simulink model "Target_Control_System"  (R2021b)
settings: Solver=FixedStepDiscrete  StartTime=0.0  StopTime=5  RelTol=1e-3
PreLoadFcn:
  | RTWConfigurationCB('preloadfcn', bdroot);
PostLoadFcn:
  | load('configuration/data_struct.mat');
  | load('configuration/fluxMaps_propMotor.mat');
  | load('configuration/parameterInit_PROP.mat');
  | load('configuration/parameterInit_PUMP.mat');
  | load('configuration/parameterInit_PITCH.mat');
  | load('configuration/parameterInit_TILT.mat');
  | %load('configuration/base_workspace_signal_definition.mat');
  | %load('resolvedatastores_to_baseworkspace_for_faster_simulation.mat');
model workspace (MAT data in the model file):
  SIMULATION_OPTIONS : Simulink.Parameter (value not decoded)
  TARGET_CODE_GEN : Simulink.Parameter (value not decoded)
  TCS_SAMPLE_FREQ_HZ : Simulink.Parameter (value not decoded)
symbols that are objects in the model workspace (value not decoded): TARGET_CODE_GEN, TCS_SAMPLE_FREQ_HZ
undefined symbols (not defined in the file): A_DQ_REF_LPF_INIT__PITCH, A_DQ_REF_LPF_INIT__PROP, A_DQ_REF_LPF_INIT__PUMP, A_DQ_REF_LPF_INIT__TILT, A_OBSERVER_CONFIDENCE_INIT__PITCH, A_OBSERVER_CONFIDENCE_INIT__PROP, A_OBSERVER_CONFIDENCE_INIT__PUMP, A_OBSERVER_CONFIDENCE_INIT__TILT, ACTUATOR_MAX_ANGLE_TRIP__PITCH, ACTUATOR_MIN_ANGLE_TRIP__PITCH, ACTUATOR_POS_SENSOR_INV_DIRECTION__PITCH, ACTUATOR_POS_SENSOR_INV_DIRECTION__TILT, ACTUATOR_POS_SENSOR_OFFSET__PITCH, ACTUATOR_POS_SENSOR_OFFSET__TILT, ADC_scaler1_baseaddr_TILT, ADC_SCALER_FLOAT_TO_FIXPOINT_EXPANSION, ANGLE_ELEC_FROM_SENSOR_OFFSET_INIT__PITCH, ANGLE_ELEC_FROM_SENSOR_OFFSET_INIT__PROP, ANGLE_ELEC_FROM_SENSOR_OFFSET_INIT__PUMP, ANGLE_ELEC_FROM_SENSOR_OFFSET_INIT__TILT, AUTO_CLEAR_FAULTS_ENABLED__PITCH, AUTO_CLEAR_FAULTS_ENABLED__PROP, AUTO_CLEAR_FAULTS_ENABLED__PUMP, AUTO_CLEAR_FAULTS_ENABLED__TILT, AUTO_CLEAR_FAULTS_WAIT_TICKS__PITCH, AUTO_CLEAR_FAULTS_WAIT_TICKS__PROP, AUTO_CLEAR_FAULTS_WAIT_TICKS__PUMP, AUTO_CLEAR_FAULTS_WAIT_TICKS__TILT, AUTO_I_ZERO_IDLE_TICKS__PITCH, AUTO_I_ZERO_IDLE_TICKS__PROP, AUTO_I_ZERO_IDLE_TICKS__PUMP, AUTO_I_ZERO_IDLE_TICKS__TILT, AUTO_I_ZERO_OFFSET_IDC_THRESHOLD__PITCH, AUTO_I_ZERO_OFFSET_IDC_THRESHOLD__PROP, AUTO_I_ZERO_OFFSET_IDC_THRESHOLD__PUMP, AUTO_I_ZERO_OFFSET_IDC_THRESHOLD__TILT, AUTO_I_ZERO_OFFSET_IPH_THRESHOLD__PITCH, AUTO_I_ZERO_OFFSET_IPH_THRESHOLD__PROP, AUTO_I_ZERO_OFFSET_IPH_THRESHOLD__PUMP, AUTO_I_ZERO_OFFSET_IPH_THRESHOLD__TILT, AUTO_SENSORLESS_SWITCHOVER_DISABLE_OMEGA, AUTO_SENSORLESS_SWITCHOVER_ENABLE_OMEGA, AUTO_SENSORLESS_SWITCHOVER_MIN_CONFIDENCE, AUXILIARY_PROTECTION_UNIT_BASEADDR__TILT, blanking_max_error_omega_INIT_PITCH, blanking_max_error_omega_INIT_TILT, blanking_max_error_position_INIT_PITCH, blanking_max_error_position_INIT_TILT, BRUTE_START_I_Q_REF_RAMP_SPEED__PITCH, BRUTE_START_I_Q_REF_RAMP_SPEED__PROP, BRUTE_START_I_Q_REF_RAMP_SPEED__PUMP, BRUTE_START_I_Q_REF_RAMP_SPEED__TILT, CONTROL_LOOP_DT_INIT__PITCH, CONTROL_LOOP_DT_INIT__PROP, CONTROL_LOOP_DT_INIT__PUMP, CONTROL_LOOP_DT_INIT__TILT, CORRECTION_FILTER_SCALE__PITCH, CORRECTION_FILTER_SCALE__PROP, CORRECTION_FILTER_SCALE__PUMP, CORRECTION_FILTER_SCALE__TILT ... (+458)
libraries: simulink x178, Reusables_Lib x24
(part 18 of 47)

== system Target_Control_System/Target_Control_System/Simulation Controls/Simulation Data Store Initialization/initializeDataForTilt()/initializeHardwareInvTilt ==
  initializeHardwareInvTilt : TriggerPort  TriggerType=function-call  VariantControl=Variant
  Constant : Constant  Value=4.0  OutDataTypeStr=single
  Constant1 : Constant  Value=DEADTIME_NS__TILT  OutDataTypeStr=single
  Constant10 : Constant  Value=VOLTAGE_OFFSET_DC_V_JULY2019__TILT  OutDataTypeStr=single
  Constant11 : Constant  Value=FULL_SCALE_VALUE_DC_VOLTAGE_V_JULY2019__TILT  OutDataTypeStr=single
  Constant12 : Constant  Value=ADC_SCALER_FLOAT_TO_FIXPOINT_EXPANSION  OutDataTypeStr=single
  Constant13 : Constant  Value=PHASE_CURRENT_SUM_MAX_IMBALANCE__TILT  OutDataTypeStr=single
  Constant14 : Constant  Value=MAX_IDENTICAL_SAMPLES_PHASE_CURRENT__TILT  OutDataTypeStr=int32
  Constant15 : Constant  Value=AUXILIARY_PROTECTION_UNIT_BASEADDR__TILT  OutDataTypeStr=uint32
  Constant16 : Constant  Commented=on  Value=GateDriver_baseaddr_TILT  OutDataTypeStr=single
  Constant17 : Constant  Commented=on  Value=ADC_scaler1_baseaddr_TILT  OutDataTypeStr=single
  Constant18 : Constant  Commented=on  Value=PWM1_baseaddr_TILT  OutDataTypeStr=single
  Constant19 : Constant  Commented=on  Value=IIR_baseaddr_TILT  OutDataTypeStr=single
  Constant2 : Constant  Value=IIR_DC_F_INIT__TILT  OutDataTypeStr=single
  Constant21 : Constant  Commented=on  Value=TILT_INPUT_ENCODER_base_addr  OutDataTypeStr=single
  Constant22 : Constant  Commented=on  Value=TILT_OUTPUT_ENCODER_base_addr  OutDataTypeStr=single
  Constant3 : Constant  Value=IIR_UPHASE_F_INIT__TILT  OutDataTypeStr=single
  Constant4 : Constant  Value=IIR_IPHASE_F_INIT__TILT  OutDataTypeStr=single
  Constant5 : Constant  Value=IIR_F_SAMPLE__TILT  OutDataTypeStr=single
  Constant6 : Constant  Value=FULL_SCALE_VALUE_PHASE_VOLTAGE_V__TILT  OutDataTypeStr=single
  Constant7 : Constant  Value=FULL_SCALE_VALUE_PHASE_CURRENT_A__TILT  OutDataTypeStr=single
  Constant8 : Constant  Value=FULL_SCALE_VALUE_DC_CURRENT_A__TILT  OutDataTypeStr=single
  Constant9 : Constant  Value=VOLTAGE_OFFSET_V__TILT  OutDataTypeStr=single
  Data Store Write : DataStoreWrite  DataStoreName=oTilt  DataStoreElements=oTilt.oHw_.fTripLimitHardware_  IndexOptions=Index vector (dialog)  Indices=1  OutputSizes=1
  Data Store Write1 : DataStoreWrite  DataStoreName=oTilt  DataStoreElements=oTilt.oHw_.fDeadtimeNs_  IndexOptions=Index vector (dialog)  Indices=1  OutputSizes=1
  Data Store Write10 : DataStoreWrite  DataStoreName=oTilt  DataStoreElements=oTilt.oHw_.fFullScaleValueDcVoltage_  IndexOptions=Index vector (dialog)  Indices=1  OutputSizes=1
  Data Store Write11 : DataStoreWrite  DataStoreName=oTilt  DataStoreElements=oTilt.oHw_.fVoltageOffsetDcInVolts_  IndexOptions=Index vector (dialog)  Indices=1  OutputSizes=1
  Data Store Write12 : DataStoreWrite  DataStoreName=oTilt  DataStoreElements=oTilt.oHw_.iScalePhaseCurrentLong_  IndexOptions=Index vector (dialog)  Indices=1  OutputSizes=1
  Data Store Write13 : DataStoreWrite  DataStoreName=oTilt  DataStoreElements=oTilt.oHw_.iScaleDcCurrentLong_  IndexOptions=Index vector (dialog)  Indices=1  OutputSizes=1
  Data Store Write14 : DataStoreWrite  DataStoreName=oTilt  DataStoreElements=oTilt.oHw_.iScalePhaseVoltageLong_  IndexOptions=Index vector (dialog)  Indices=1  OutputSizes=1
  Data Store Write15 : DataStoreWrite  DataStoreName=oTilt  DataStoreElements=oTilt.oHw_.iScaleDcVoltageLong_  IndexOptions=Index vector (dialog)  Indices=1  OutputSizes=1
  Data Store Write16 : DataStoreWrite  DataStoreName=oTilt  DataStoreElements=oTilt.oHw_.fPhaseCurrentSumMaxImbalance_  IndexOptions=Index vector (dialog)  Indices=1  OutputSizes=1
  Data Store Write17 : DataStoreWrite  DataStoreName=oTilt  DataStoreElements=oTilt.oHw_.iMaxIdenticalSamplesPhaseCurrent_  IndexOptions=Index vector (dialog)  Indices=1  OutputSizes=1
  Data Store Write18 : DataStoreWrite  DataStoreName=oTilt  DataStoreElements=oTilt.oHw_.uiAuxiliaryProtectionUnitBaseaddr_  IndexOptions=Index vector (dialog)  Indices=1  OutputSizes=1
  Data Store Write19 : DataStoreWrite  DataStoreName=oTilt  DataStoreElements=oTilt.oHw_.iVoltageOffsetPhsLong_  IndexOptions=Index vector (dialog)  Indices=1  OutputSizes=1
  Data Store Write2 : DataStoreWrite  DataStoreName=oTilt  DataStoreElements=oTilt.oHw_.fIirDcFInit_  IndexOptions=Index vector (dialog)  Indices=1  OutputSizes=1
  Data Store Write20 : DataStoreWrite  DataStoreName=oTilt  DataStoreElements=oTilt.oHw_.iVoltageOffsetDcLong_  IndexOptions=Index vector (dialog)  Indices=1  OutputSizes=1
  Data Store Write21 : DataStoreWrite  Commented=on  DataStoreName=oTilt  DataStoreElements=oTilt.oHw_.uiPwmGeneratorBaseaddr_  IndexOptions=Index vector (dialog)  Indices=1  OutputSizes=1
  Data Store Write22 : DataStoreWrite  Commented=on  DataStoreName=oTilt  DataStoreElements=oTilt.oHw_.uiIirInterfaceBaseaddr_  IndexOptions=Index vector (dialog)  Indices=1  OutputSizes=1
  Data Store Write23 : DataStoreWrite  Commented=on  DataStoreName=oTilt  DataStoreElements=oTilt.oHw_.uiInputPositionSensorBaseaddr_  IndexOptions=Index vector (dialog)  Indices=1  OutputSizes=1
  Data Store Write24 : DataStoreWrite  Commented=on  DataStoreName=oTilt  DataStoreElements=oTilt.oHw_.uiOutputPositionSensorBaseaddr_  IndexOptions=Index vector (dialog)  Indices=1  OutputSizes=1
  Data Store Write26 : DataStoreWrite  Commented=on  DataStoreName=oTilt  DataStoreElements=oTilt.oHw_.uiGateDriverBaseaddr_  IndexOptions=Index vector (dialog)  Indices=1  OutputSizes=1
  Data Store Write27 : DataStoreWrite  Commented=on  DataStoreName=oTilt  DataStoreElements=oTilt.oHw_.uiAdcScalerBaseaddr_  IndexOptions=Index vector (dialog)  Indices=1  OutputSizes=1
  Data Store Write3 : DataStoreWrite  DataStoreName=oTilt  DataStoreElements=oTilt.oHw_.fIirUphaseFInit_  IndexOptions=Index vector (dialog)  Indices=1  OutputSizes=1
  Data Store Write4 : DataStoreWrite  DataStoreName=oTilt  DataStoreElements=oTilt.oHw_.fIirIphaseFInit_  IndexOptions=Index vector (dialog)  Indices=1  OutputSizes=1
  Data Store Write5 : DataStoreWrite  DataStoreName=oTilt  DataStoreElements=oTilt.oHw_.fIirFSample_  IndexOptions=Index vector (dialog)  Indices=1  OutputSizes=1
  Data Store Write6 : DataStoreWrite  DataStoreName=oTilt  DataStoreElements=oTilt.oHw_.fFullScaleValuePhaseCurrent_  IndexOptions=Index vector (dialog)  Indices=1  OutputSizes=1
  Data Store Write7 : DataStoreWrite  DataStoreName=oTilt  DataStoreElements=oTilt.oHw_.fFullScaleValueDcCurrent_  IndexOptions=Index vector (dialog)  Indices=1  OutputSizes=1
  Data Store Write8 : DataStoreWrite  DataStoreName=oTilt  DataStoreElements=oTilt.oHw_.fFullScaleValuePhaseVoltage_  IndexOptions=Index vector (dialog)  Indices=1  OutputSizes=1
  Data Store Write9 : DataStoreWrite  DataStoreName=oTilt  DataStoreElements=oTilt.oHw_.fVoltageOffsetInVolts_  IndexOptions=Index vector (dialog)  Indices=1  OutputSizes=1
  Divide{,1..5} (6 alike) : Product  Inputs=**  OutDataTypeStr=int32
  wires:
  Divide1/1 -> Data Store Write12/1
  Divide/1 -> Data Store Write13/1
  Constant10/1 -> Data Store Write11/1, Divide5/1
  Divide5/1 -> Data Store Write20/1
  Divide4/1 -> Data Store Write19/1
  Constant9/1 -> Data Store Write9/1, Divide4/1
  Constant22/1 -> Data Store Write24/1
  Constant4/1 -> Data Store Write4/1
  Constant3/1 -> Data Store Write3/1
  Constant2/1 -> Data Store Write2/1
  Constant17/1 -> Data Store Write27/1
  Constant8/1 -> Data Store Write7/1, Divide/1
  Divide2/1 -> Data Store Write14/1
  Divide3/1 -> Data Store Write15/1
  Constant1/1 -> Data Store Write1/1
  Constant11/1 -> Data Store Write10/1, Divide3/1
  Constant15/1 -> Data Store Write18/1
  Constant5/1 -> Data Store Write5/1
  Constant6/1 -> Data Store Write8/1, Divide2/1
  Constant14/1 -> Data Store Write17/1
  Constant19/1 -> Data Store Write22/1
  Constant/1 -> Data Store Write/1
  Constant18/1 -> Data Store Write21/1
  Constant16/1 -> Data Store Write26/1
  Constant12/1 -> Divide/2, Divide5/2, Divide3/2, Divide4/2, Divide2/2, Divide1/2
  Constant13/1 -> Data Store Write16/1
  Constant21/1 -> Data Store Write23/1
  Constant7/1 -> Data Store Write6/1, Divide1/1

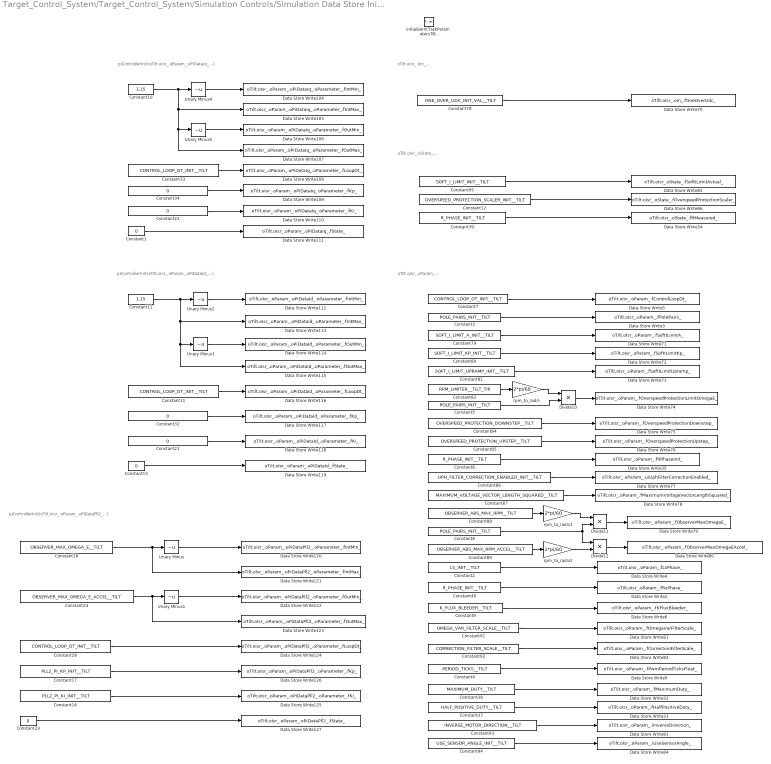
== system Target_Control_System/Target_Control_System/Simulation Controls/Simulation Data Store Initialization/initializeDataForTilt()/initializeIntTaskParametersTilt ==
  note: oTilt.oIsr_.oState_...
  note: oTilt.oIsr_.oParam_...
  note: oTilt.oIsr_.oIn_...
  note: piControllerInit(oTilt.oIsr_.oParam_.oPiDataIq_...)
  note: piControllerInit(oTilt.oIsr_.oParam_.oPiDataPll2_...)
  note: piControllerInit(oTilt.oIsr_.oParam_.oPiDataId_...)
  initializeIntTaskParametersTilt : TriggerPort  TriggerType=function-call  VariantControl=Variant
  Constant{1,15,21..22,32,34} (6 alike) : Constant  Value=0  OutDataTypeStr=single  SampleTime=-1
  Constant10 : Constant  Value=1.15  OutDataTypeStr=single  SampleTime=-1
  Constant11 : Constant  Value=1.15  OutDataTypeStr=single  SampleTime=-1
  Constant12 : Constant  Value=OVERSPEED_PROTECTION_SCALER_INIT__TILT  OutDataTypeStr=single  SampleTime=-1
  Constant16 : Constant  Value=PLL2_PI_KI_INIT__TILT  OutDataTypeStr=single  SampleTime=-1
  Constant17 : Constant  Value=PLL2_PI_KP_INIT__TILT  OutDataTypeStr=single  SampleTime=-1
  Constant18 : Constant  Value=OBSERVER_MAX_OMEGA_E__TILT  OutDataTypeStr=single  SampleTime=-1
  Constant2 : Constant  Value=LS_INIT__TILT  OutDataTypeStr=single  SampleTime=-1
  Constant23 : Constant  Value=0  OutDataTypeStr=single
  Constant24 : Constant  Value=OBSERVER_MAX_OMEGA_E_ACCEL__TILT  OutDataTypeStr=single  SampleTime=-1
  Constant28 : Constant  Value=CONTROL_LOOP_DT_INIT__TILT  OutDataTypeStr=single  SampleTime=-1
  Constant3 : Constant  Value=POLE_PAIRS_INIT__TILT  VectorParams1D=off  OutDataTypeStr=single  SampleTime=-1
  Constant31 : Constant  Value=CONTROL_LOOP_DT_INIT__TILT  OutDataTypeStr=single  SampleTime=-1
  Constant33 : Constant  Value=CONTROL_LOOP_DT_INIT__TILT  OutDataTypeStr=single  SampleTime=-1
  Constant37 : Constant  Value=HALF_POSITIVE_DUTY__TILT  OutDataTypeStr=single  SampleTime=-1
  Constant38 : Constant  Value=MAXIMUM_DUTY__TILT  OutDataTypeStr=single  SampleTime=-1
  Constant39 : Constant  Value=R_PHASE_INIT__TILT  OutDataTypeStr=single  SampleTime=-1
  Constant4 : Constant  Value=PERIOD_TICKS__TILT  OutDataTypeStr=single  SampleTime=-1
  Constant40 : Constant  Value=R_PHASE_INIT__TILT  OutDataTypeStr=single  SampleTime=-1
  Constant5 : Constant  Value=POLE_PAIRS_INIT__TILT  VectorParams1D=off  OutDataTypeStr=single  SampleTime=-1
  Constant6 : Constant  Value=R_PHASE_INIT__TILT  VectorParams1D=off  OutDataTypeStr=single  SampleTime=-1
  Constant7 : Constant  Value=CONTROL_LOOP_DT_INIT__TILT  VectorParams1D=off  OutDataTypeStr=single  SampleTime=-1
  Constant78 : Constant  Value=ONE_OVER_UDC_INIT_VAL__TILT  VectorParams1D=off  OutDataTypeStr=single  SampleTime=-1
  Constant79 : Constant  Value=SOFT_I_LIMIT_A_INIT__TILT  OutDataTypeStr=single  SampleTime=-1
  Constant8 : Constant  Value=POLE_PAIRS_INIT__TILT  VectorParams1D=off  OutDataTypeStr=single  SampleTime=-1
  Constant80 : Constant  Value=SOFT_I_LIMIT_KP_INIT__TILT  OutDataTypeStr=single  SampleTime=-1
  Constant81 : Constant  Value=SOFT_I_LIMIT_UPRAMP_INIT__TILT  OutDataTypeStr=single  SampleTime=-1
  Constant82 : Constant  Value=RPM_LIMITER__TILT_TIP  OutDataTypeStr=single  SampleTime=-1
  Constant84 : Constant  Value=OVERSPEED_PROTECTION_DOWNSTEP__TILT  OutDataTypeStr=single  SampleTime=-1
  Constant85 : Constant  Value=OVERSPEED_PROTECTION_UPSTEP__TILT  OutDataTypeStr=single  SampleTime=-1
  Constant86 : Constant  Value=UPH_FILTER_CORRECTION_ENABLED_INIT__TILT  OutDataTypeStr=uint32  SampleTime=-1
  Constant87 : Constant  Value=MAXIMUM_VOLTAGE_VECTOR_LENGTH_SQUARED__TILT  VectorParams1D=off  OutDataTypeStr=single  SampleTime=-1
  Constant88 : Constant  Value=OBSERVER_ABS_MAX_RPM__TILT  OutDataTypeStr=single  SampleTime=-1
  Constant89 : Constant  Value=OBSERVER_ABS_MAX_RPM_ACCEL__TILT  OutDataTypeStr=single  SampleTime=-1
  Constant9 : Constant  Value=K_FLUX_BLEEDER__TILT  VectorParams1D=off  OutDataTypeStr=single  SampleTime=-1
  Constant91 : Constant  Value=OMEGA_VAR_FILTER_SCALE__TILT  OutDataTypeStr=single  SampleTime=-1
  Constant92 : Constant  Value=CORRECTION_FILTER_SCALE__TILT  OutDataTypeStr=single  SampleTime=-1
  Constant93 : Constant  Value=INVERSE_MOTOR_DIRECTION__TILT  OutDataTypeStr=int32  SampleTime=-1
  Constant94 : Constant  Value=USE_SENSOR_ANGLE_INIT__TILT  OutDataTypeStr=int32  SampleTime=-1
  Constant95 : Constant  Value=SOFT_I_LIMIT_INIT__TILT  OutDataTypeStr=single  SampleTime=-1
  Data Store Write104 : DataStoreWrite  DataStoreName=oTilt  DataStoreElements=oTilt.oIsr_.oParam_.oPiDataIq_.oParameter_.fIntMin_  IndexOptions=Index vector (dialog)  Indices=1  OutputSizes=1
  Data Store Write105 : DataStoreWrite  DataStoreName=oTilt  DataStoreElements=oTilt.oIsr_.oParam_.oPiDataIq_.oParameter_.fIntMax_  IndexOptions=Index vector (dialog)  Indices=1  OutputSizes=1
  Data Store Write106 : DataStoreWrite  DataStoreName=oTilt  DataStoreElements=oTilt.oIsr_.oParam_.oPiDataIq_.oParameter_.fOutMin_  IndexOptions=Index vector (dialog)  Indices=1  OutputSizes=1
  Data Store Write107 : DataStoreWrite  DataStoreName=oTilt  DataStoreElements=oTilt.oIsr_.oParam_.oPiDataIq_.oParameter_.fOutMax_  IndexOptions=Index vector (dialog)  Indices=1  OutputSizes=1
  Data Store Write108 : DataStoreWrite  DataStoreName=oTilt  DataStoreElements=oTilt.oIsr_.oParam_.oPiDataIq_.oParameter_.fLoopDt_  IndexOptions=Index vector (dialog)  Indices=1  OutputSizes=1
  Data Store Write109 : DataStoreWrite  DataStoreName=oTilt  DataStoreElements=oTilt.oIsr_.oParam_.oPiDataIq_.oParameter_.fKp_  IndexOptions=Index vector (dialog)  Indices=1  OutputSizes=1
  Data Store Write110 : DataStoreWrite  DataStoreName=oTilt  DataStoreElements=oTilt.oIsr_.oParam_.oPiDataIq_.oParameter_.fKi_  IndexOptions=Index vector (dialog)  Indices=1  OutputSizes=1
  Data Store Write111 : DataStoreWrite  DataStoreName=oTilt  DataStoreElements=oTilt.oIsr_.oParam_.oPiDataIq_.fState_  IndexOptions=Index vector (dialog)  Indices=1  OutputSizes=1
  Data Store Write112 : DataStoreWrite  DataStoreName=oTilt  DataStoreElements=oTilt.oIsr_.oParam_.oPiDataId_.oParameter_.fIntMin_  IndexOptions=Index vector (dialog)  Indices=1  OutputSizes=1
  Data Store Write113 : DataStoreWrite  DataStoreName=oTilt  DataStoreElements=oTilt.oIsr_.oParam_.oPiDataId_.oParameter_.fIntMax_  IndexOptions=Index vector (dialog)  Indices=1  OutputSizes=1
  Data Store Write114 : DataStoreWrite  DataStoreName=oTilt  DataStoreElements=oTilt.oIsr_.oParam_.oPiDataId_.oParameter_.fOutMin_  IndexOptions=Index vector (dialog)  Indices=1  OutputSizes=1
  Data Store Write115 : DataStoreWrite  DataStoreName=oTilt  DataStoreElements=oTilt.oIsr_.oParam_.oPiDataId_.oParameter_.fOutMax_  IndexOptions=Index vector (dialog)  Indices=1  OutputSizes=1
  Data Store Write116 : DataStoreWrite  DataStoreName=oTilt  DataStoreElements=oTilt.oIsr_.oParam_.oPiDataId_.oParameter_.fLoopDt_  IndexOptions=Index vector (dialog)  Indices=1  OutputSizes=1
  Data Store Write117 : DataStoreWrite  DataStoreName=oTilt  DataStoreElements=oTilt.oIsr_.oParam_.oPiDataId_.oParameter_.fKp_  IndexOptions=Index vector (dialog)  Indices=1  OutputSizes=1
  Data Store Write118 : DataStoreWrite  DataStoreName=oTilt  DataStoreElements=oTilt.oIsr_.oParam_.oPiDataId_.oParameter_.fKi_  IndexOptions=Index vector (dialog)  Indices=1  OutputSizes=1
  Data Store Write119 : DataStoreWrite  DataStoreName=oTilt  DataStoreElements=oTilt.oIsr_.oParam_.oPiDataId_.fState_  IndexOptions=Index vector (dialog)  Indices=1  OutputSizes=1
  Data Store Write120 : DataStoreWrite  DataStoreName=oTilt  DataStoreElements=oTilt.oIsr_.oParam_.oPiDataPll2_.oParameter_.fIntMin_  IndexOptions=Index vector (dialog)  Indices=1  OutputSizes=1
  Data Store Write121 : DataStoreWrite  DataStoreName=oTilt  DataStoreElements=oTilt.oIsr_.oParam_.oPiDataPll2_.oParameter_.fIntMax_  IndexOptions=Index vector (dialog)  Indices=1  OutputSizes=1
  Data Store Write122 : DataStoreWrite  DataStoreName=oTilt  DataStoreElements=oTilt.oIsr_.oParam_.oPiDataPll2_.oParameter_.fOutMin_  IndexOptions=Index vector (dialog)  Indices=1  OutputSizes=1
  Data Store Write123 : DataStoreWrite  DataStoreName=oTilt  DataStoreElements=oTilt.oIsr_.oParam_.oPiDataPll2_.oParameter_.fOutMax_  IndexOptions=Index vector (dialog)  Indices=1  OutputSizes=1
  Data Store Write124 : DataStoreWrite  DataStoreName=oTilt  DataStoreElements=oTilt.oIsr_.oParam_.oPiDataPll2_.oParameter_.fLoopDt_  IndexOptions=Index vector (dialog)  Indices=1  OutputSizes=1
  Data Store Write125 : DataStoreWrite  DataStoreName=oTilt  DataStoreElements=oTilt.oIsr_.oParam_.oPiDataPll2_.oParameter_.fKi_  IndexOptions=Index vector (dialog)  Indices=1  OutputSizes=1
  Data Store Write126 : DataStoreWrite  DataStoreName=oTilt  DataStoreElements=oTilt.oIsr_.oParam_.oPiDataPll2_.oParameter_.fKp_  IndexOptions=Index vector (dialog)  Indices=1  OutputSizes=1
  Data Store Write127 : DataStoreWrite  DataStoreName=oTilt  DataStoreElements=oTilt.oIsr_.oParam_.oPiDataPll2_.fState_  IndexOptions=Index vector (dialog)  Indices=1  OutputSizes=1
  Data Store Write2 : DataStoreWrite  DataStoreName=oTilt  DataStoreElements=oTilt.oIsr_.oParam_.fRsPhase_  IndexOptions=Index vector (dialog)  Indices=1  OutputSizes=1
  Data Store Write3 : DataStoreWrite  DataStoreName=oTilt  DataStoreElements=oTilt.oIsr_.oParam_.fPolePairs_  IndexOptions=Index vector (dialog)  Indices=1  OutputSizes=1
  Data Store Write32 : DataStoreWrite  DataStoreName=oTilt  DataStoreElements=oTilt.oIsr_.oParam_.fMaximumDuty_  IndexOptions=Index vector (dialog)  Indices=1  OutputSizes=1
  Data Store Write33 : DataStoreWrite  DataStoreName=oTilt  DataStoreElements=oTilt.oIsr_.oParam_.fHalfPositiveDuty_  IndexOptions=Index vector (dialog)  Indices=1  OutputSizes=1
  Data Store Write34 : DataStoreWrite  DataStoreName=oTilt  DataStoreElements=oTilt.oIsr_.oState_.fRMeasured_  IndexOptions=Index vector (dialog)  Indices=1  OutputSizes=1
  Data Store Write35 : DataStoreWrite  DataStoreName=oTilt  DataStoreElements=oTilt.oIsr_.oParam_.fRPhaseInit_  IndexOptions=Index vector (dialog)  Indices=1  OutputSizes=1
  Data Store Write4 : DataStoreWrite  DataStoreName=oTilt  DataStoreElements=oTilt.oIsr_.oParam_.fLsPhase_  IndexOptions=Index vector (dialog)  Indices=1  OutputSizes=1
  Data Store Write5 : DataStoreWrite  DataStoreName=oTilt  DataStoreElements=oTilt.oIsr_.oParam_.fControlLoopDt_  IndexOptions=Index vector (dialog)  Indices=1  OutputSizes=1
  Data Store Write6 : DataStoreWrite  DataStoreName=oTilt  DataStoreElements=oTilt.oIsr_.oParam_.fKFluxBleeder_  IndexOptions=Index vector (dialog)  Indices=1  OutputSizes=1
  Data Store Write70 : DataStoreWrite  DataStoreName=oTilt  DataStoreElements=oTilt.oIsr_.oIn_.fOneOverUdc_  IndexOptions=Index vector (dialog)  Indices=1  OutputSizes=1
  Data Store Write71 : DataStoreWrite  DataStoreName=oTilt  DataStoreElements=oTilt.oIsr_.oParam_.fSoftILimitA_  IndexOptions=Index vector (dialog)  Indices=1  OutputSizes=1
  Data Store Write72 : DataStoreWrite  DataStoreName=oTilt  DataStoreElements=oTilt.oIsr_.oParam_.fSoftILimitKp_  IndexOptions=Index vector (dialog)  Indices=1  OutputSizes=1
  Data Store Write73 : DataStoreWrite  DataStoreName=oTilt  DataStoreElements=oTilt.oIsr_.oParam_.fSoftILimitUpramp_  IndexOptions=Index vector (dialog)  Indices=1  OutputSizes=1
  Data Store Write74 : DataStoreWrite  DataStoreName=oTilt  DataStoreElements=oTilt.oIsr_.oParam_.fOverspeedProtectionLimitOmegaE_  IndexOptions=Index vector (dialog)  Indices=1  OutputSizes=1
  Data Store Write75 : DataStoreWrite  DataStoreName=oTilt  DataStoreElements=oTilt.oIsr_.oParam_.fOverspeedProtectionDownstep_  IndexOptions=Index vector (dialog)  Indices=1  OutputSizes=1
  Data Store Write76 : DataStoreWrite  DataStoreName=oTilt  DataStoreElements=oTilt.oIsr_.oParam_.fOverspeedProtectionUpstep_  IndexOptions=Index vector (dialog)  Indices=1  OutputSizes=1
  Data Store Write77 : DataStoreWrite  DataStoreName=oTilt  DataStoreElements=oTilt.oIsr_.oParam_.uiUphFilterCorrectionEnabled_  IndexOptions=Index vector (dialog)  Indices=1  OutputSizes=1
  Data Store Write78 : DataStoreWrite  DataStoreName=oTilt  DataStoreElements=oTilt.oIsr_.oParam_.fMaximumVoltageVectorLengthSquared_  IndexOptions=Index vector (dialog)  Indices=1  OutputSizes=1
  Data Store Write79 : DataStoreWrite  DataStoreName=oTilt  DataStoreElements=oTilt.oIsr_.oParam_.fObserverMaxOmegaE_  IndexOptions=Index vector (dialog)  Indices=1  OutputSizes=1
  Data Store Write80 : DataStoreWrite  DataStoreName=oTilt  DataStoreElements=oTilt.oIsr_.oParam_.fObserverMaxOmegaEAccel_  IndexOptions=Index vector (dialog)  Indices=1  OutputSizes=1
  Data Store Write81 : DataStoreWrite  DataStoreName=oTilt  DataStoreElements=oTilt.oIsr_.oParam_.fOmegaVarFilterScale_  IndexOptions=Index vector (dialog)  Indices=1  OutputSizes=1
  Data Store Write82 : DataStoreWrite  DataStoreName=oTilt  DataStoreElements=oTilt.oIsr_.oParam_.fCorrectionFilterScale_  IndexOptions=Index vector (dialog)  Indices=1  OutputSizes=1
  Data Store Write83 : DataStoreWrite  DataStoreName=oTilt  DataStoreElements=oTilt.oIsr_.oParam_.iInverseDirection_  IndexOptions=Index vector (dialog)  Indices=1  OutputSizes=1
  Data Store Write84 : DataStoreWrite  DataStoreName=oTilt  DataStoreElements=oTilt.oIsr_.oParam_.iUseSensorAngle_  IndexOptions=Index vector (dialog)  Indices=1  OutputSizes=1
  Data Store Write85 : DataStoreWrite  DataStoreName=oTilt  DataStoreElements=oTilt.oIsr_.oState_.fSoftILimitActual_  IndexOptions=Index vector (dialog)  Indices=1  OutputSizes=1
  Data Store Write86 : DataStoreWrite  DataStoreName=oTilt  DataStoreElements=oTilt.oIsr_.oState_.fOverspeedProtectionScaler_  IndexOptions=Index vector (dialog)  Indices=1  OutputSizes=1
  Data Store Write9 : DataStoreWrite  DataStoreName=oTilt  DataStoreElements=oTilt.oIsr_.oParam_.fPwmPeriodTicksFloat_  IndexOptions=Index vector (dialog)  Indices=1  OutputSizes=1
  Divide10 : Product  Inputs=**
  Divide11 : Product  Inputs=**
  Divide12 : Product  Inputs=**
  Unary Minus{,1..5} (6 alike) : UnaryMinus
  rpm_to_rad/s : Gain  Gain=2*pi/60
  rpm_to_rad/s1 : Gain  Gain=2*pi/60
  rpm_to_rad/s2 : Gain  Gain=2*pi/60
  wires:
  Constant39/1 -> Data Store Write34/1
  Constant12/1 -> Data Store Write86/1
  Constant95/1 -> Data Store Write85/1
  Constant8/1 -> Divide11/2, Divide12/1
  Constant5/1 -> Divide10/2
  Constant6/1 -> Data Store Write35/1
  Divide10/1 -> Data Store Write74/1
  Constant88/1 -> rpm_to_rad/s1/1
  Constant3/1 -> Data Store Write3/1
  Constant9/1 -> Data Store Write6/1
  Constant7/1 -> Data Store Write5/1
  Divide11/1 -> Data Store Write79/1
  Constant40/1 -> Data Store Write2/1
  Constant81/1 -> Data Store Write73/1
  Constant82/1 -> rpm_to_rad/s/1
  Constant84/1 -> Data Store Write75/1
  Constant4/1 -> Data Store Write9/1
  Constant86/1 -> Data Store Write77/1
  Constant87/1 -> Data Store Write78/1
  Constant91/1 -> Data Store Write81/1
  Constant94/1 -> Data Store Write84/1
  rpm_to_rad/s2/1 -> Divide12/2
  Constant93/1 -> Data Store Write83/1
  Constant2/1 -> Data Store Write4/1
  Constant38/1 -> Data Store Write32/1
  Constant37/1 -> Data Store Write33/1
  Constant89/1 -> rpm_to_rad/s2/1
  Constant85/1 -> Data Store Write76/1
  Divide12/1 -> Data Store Write80/1
  rpm_to_rad/s/1 -> Divide10/1
  Constant80/1 -> Data Store Write72/1
  Constant92/1 -> Data Store Write82/1
  Constant79/1 -> Data Store Write71/1
  rpm_to_rad/s1/1 -> Divide11/1
  Constant78/1 -> Data Store Write70/1
  Unary Minus5/1 -> Data Store Write106/1
  Unary Minus4/1 -> Data Store Write104/1
  Unary Minus3/1 -> Data Store Write114/1
  Unary Minus2/1 -> Data Store Write112/1
  Unary Minus1/1 -> Data Store Write122/1
  Unary Minus/1 -> Data Store Write120/1
  Constant1/1 -> Data Store Write111/1
  Constant17/1 -> Data Store Write126/1
  Constant21/1 -> Data Store Write118/1
  Constant24/1 -> Unary Minus1/1, Data Store Write123/1
  Constant34/1 -> Data Store Write109/1
  Constant28/1 -> Data Store Write124/1
  Constant15/1 -> Data Store Write119/1
  Constant10/1 -> Unary Minus4/1, Data Store Write105/1, Unary Minus5/1, Data Store Write107/1
  Constant32/1 -> Data Store Write117/1
  Constant31/1 -> Data Store Write116/1
  Constant33/1 -> Data Store Write108/1
  Constant11/1 -> Unary Minus2/1, Data Store Write113/1, Unary Minus3/1, Data Store Write115/1
  Constant16/1 -> Data Store Write125/1
  Constant22/1 -> Data Store Write110/1
  Constant23/1 -> Data Store Write127/1
  Constant18/1 -> Unary Minus/1, Data Store Write121/1
